simulink model "circuito_mallas"  (R2019a)
settings: Solver=VariableStepAuto  StartTime=0.0  StopTime=15  RelTol=1e-3
values from neighbouring files (symbols this model uses):
  C1 = 1e-6    (= 1e-06)    [circuito2.m]
  C2 = 200e-6    (= 0.0002)    [circuito2.m]
  L = 5e-3    (= 0.005)    [circuito2.m]
  R = 10e3    (= 10000)    [circuito2.m]
settings Model: Creator=cmparedes  LastModifiedBy=cmparedes

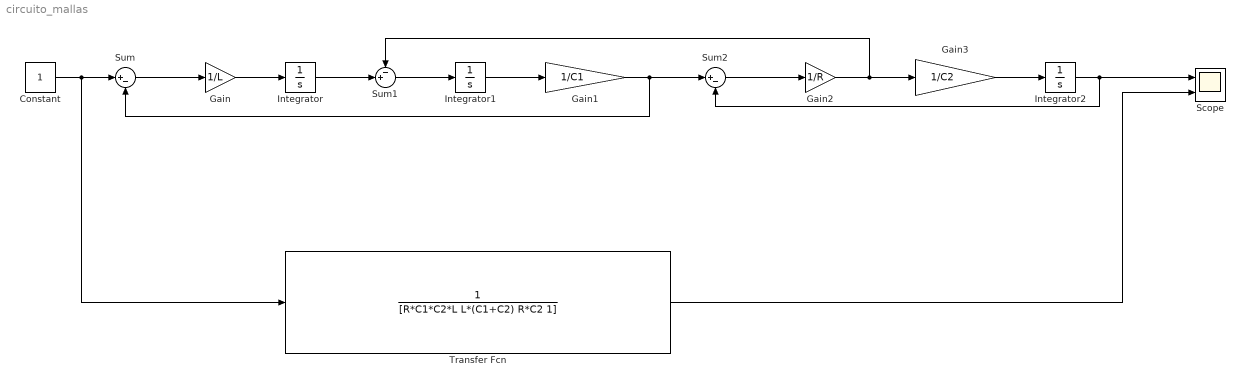
== system circuito_mallas ==
  Constant : Constant
  Gain : Gain  Gain=1/L
  Gain1 : Gain  Gain=1/C1
  Gain2 : Gain  Gain=1/R
  Gain3 : Gain  Gain=1/C2
  Integrator : Integrator
  Integrator1 : Integrator
  Integrator2 : Integrator
  Scope : Scope  NumInputPorts=2
  Sum : Sum  Inputs=|+-
  Sum1 : Sum  Inputs=-+|
  Sum2 : Sum  Inputs=|+-
  Transfer Fcn : TransferFcn  Denominator=[R*C1*C2*L L*(C1+C2) R*C2 1]
  wires:
  Sum/1 -> Gain/1
  Gain/1 -> Integrator/1
  Integrator/1 -> Sum1/2
  Sum1/1 -> Integrator1/1
  Integrator1/1 -> Gain1/1
  Gain1/1 -> Sum2/1, Sum/2
  Sum2/1 -> Gain2/1
  Gain2/1 -> Sum1/1, Gain3/1
  Gain3/1 -> Integrator2/1
  Integrator2/1 -> Scope/1, Sum2/2
  Constant/1 -> Transfer Fcn/1, Sum/1
  Transfer Fcn/1 -> Scope/2
